simulink library "fm_copter_loiter_indi_lib"  (R2018b)
settings: Solver=VariableStepAuto  StartTime=0.0  StopTime=10.0  RelTol=1e-3
undefined symbols (not defined in the file or in its folder): fm_loiter
libraries: axes_transformation_lib x1, simulink x1, cntrl_horiz_pos_indi_lib x1, fm_copter_alt_hold_indi_lib x1
settings Model: Creator=Ybeyer  LastModifiedBy=Yannic
settings SFSimCC: SimUseLocalCustomCode=off
settings RTWCC: RTWUseLocalCustomCode=off
settings CodeAppCC: StateflowObjectComments=on

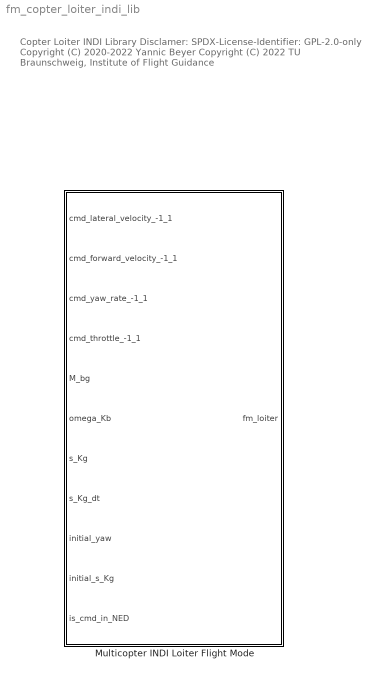
== system fm_copter_loiter_indi_lib ==
  note: Copter Loiter INDI Library
      |
      | Disclamer:
      | SPDX-License-Identifier: GPL-2.0-only
      |
      | Copyright (C) 2020-2022 Yannic Beyer
      | Copyright (C) 2022 TU Braunschweig, Institute of Flight Guidance
  Multicopter INDI Loiter Flight Mode : Subsystem  mask{fm=fm_loiter}
      mask prompts: fm "Multicopter INDI loiter flight  struct"
      mask DialogControl DescGroupVar Prompt: Multicopter INDI Loiter Flight Mode
      mask DialogControl DescTextVar Prompt: Loiter flight mode using the reduced attitude controller with INDI.
      mask DialogControl Control2 Prompt: To intialize the parameters struct see multicopterFlightModeLoiter.

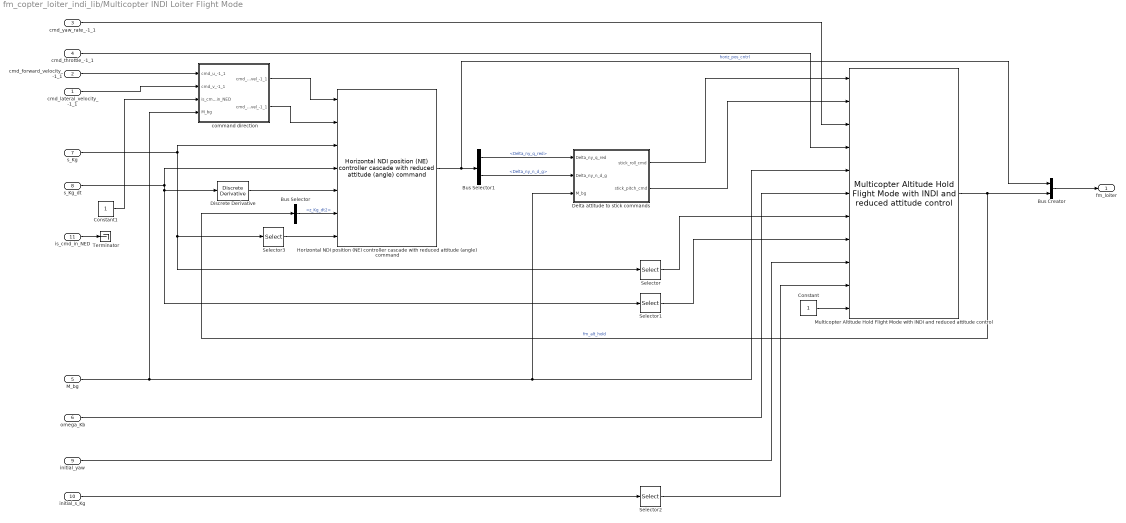
== system fm_copter_loiter_indi_lib/Multicopter INDI Loiter Flight Mode ==
  cmd_lateral_velocity_-1_1 : Inport  SampleTime=fm.sample_time
  cmd_forward_velocity_-1_1 : Inport  Port=2  SampleTime=fm.sample_time
  cmd_yaw_rate_-1_1 : Inport  Port=3  SampleTime=fm.sample_time
  cmd_throttle_-1_1 : Inport  Port=4  SampleTime=fm.sample_time
  M_bg : Inport  Port=5  SampleTime=fm.sample_time
  omega_Kb : Inport  Port=6  SampleTime=fm.sample_time
  s_Kg : Inport  Port=7  SampleTime=fm.sample_time
  s_Kg_dt : Inport  Port=8  SampleTime=fm.sample_time
  initial_yaw : Inport  Port=9  SampleTime=fm.sample_time
  initial_s_Kg : Inport  Port=10  SampleTime=fm.sample_time
  is_cmd_in_NED : Inport  Port=11  SampleTime=fm.sample_time
  Bus Creator : BusCreator  Inputs=2
  Bus Selector : BusSelector  OutputSignals=alt_cntrl.reference.z_Kg_dt2
  Bus Selector1 : BusSelector  OutputSignals=pseudo_control.Delta_ny_q_red,pseudo_control.Delta_ny_n_d_g
  Constant : Constant
  Constant1 : Constant  OutDataTypeStr=Inherit: Inherit via back propagation
  Delta attitude to stick commands : Subsystem
  Discrete Derivative : simulink/Discrete/Discrete Derivative  gainval=1.0  ICPrevScaledInput=0.0  OutMin=[]  OutMax=[]  OutDataType=fixdt(1, 16)  OutScaling=2^-10  DoSatur=off
  Horizontal NDI position (NE) controller cascade with reduced attitude (angle) command : cntrl_horiz_pos_indi_lib/Horizontal NDI position (NE) controller cascade with reduced attitude (angle) command  horiz_pos_cntrl=fm.horiz_pos_cntrl  T=2./fm.fm_alt.cntrl.atti_cntrl.rm.lean.omega + fm.fm_alt.motor_time_constant + 2./fm.fm_alt.sens_filt.omega
      settings: SourceProductName=LADAC
  Multicopter Altitude Hold Flight Mode with INDI and reduced attitude control : fm_copter_alt_hold_indi_lib/Multicopter Altitude Hold Flight Mode with INDI and reduced attitude control  fm=fm.fm_alt
      settings: SourceProductName=LADAC
  Selector : Selector  InputPortWidth=3  IndexOptions=Index vector (dialog)  Indices=3  OutputSizes=1
  Selector1 : Selector  InputPortWidth=3  IndexOptions=Index vector (dialog)  Indices=3  OutputSizes=1
  Selector2 : Selector  InputPortWidth=3  IndexOptions=Index vector (dialog)  Indices=3  OutputSizes=1
  Selector3 : Selector  InputPortWidth=3  IndexOptions=Index vector (dialog)  Indices=[1,2]  OutputSizes=1
  Terminator : Terminator
  command direction : Subsystem
  fm_loiter : Outport  OutDataTypeStr=single  SampleTime=fm.sample_time
  wires:
  cmd_forward_velocity_-1_1/1 -> command direction/1(cmd_u_-1_1)
  s_Kg_dt/1 -> Horizontal NDI position (NE) controller cascade with reduced attitude (angle) command/4, Discrete Derivative/1, Selector1/1
  Discrete Derivative/1 -> Horizontal NDI position (NE) controller cascade with reduced attitude (angle) command/5
  cmd_yaw_rate_-1_1/1 -> Multicopter Altitude Hold Flight Mode with INDI and reduced attitude control/3
  Constant/1 -> Multicopter Altitude Hold Flight Mode with INDI and reduced attitude control/11
  Selector3/1 -> Horizontal NDI position (NE) controller cascade with reduced attitude (angle) command/7
  initial_s_Kg/1 -> Selector2/1
  omega_Kb/1 -> Multicopter Altitude Hold Flight Mode with INDI and reduced attitude control/6
  Horizontal NDI position (NE) controller cascade with reduced attitude (angle) command/1 -> Bus Creator/1, Bus Selector1/1  "horiz_pos_cntrl"
  Bus Selector1/2 -> Delta attitude to stick commands/2(Delta_ny_n_d_g)  "<Delta_ny_n_d_g>"
  M_bg/1 -> Delta attitude to stick commands/3(M_bg), Multicopter Altitude Hold Flight Mode with INDI and reduced attitude control/5, command direction/4(M_bg)
  Multicopter Altitude Hold Flight Mode with INDI and reduced attitude control/1 -> Bus Creator/2, Bus Selector/1  "fm_alt_hold"
  Selector1/1 -> Multicopter Altitude Hold Flight Mode with INDI and reduced attitude control/8
  s_Kg/1 -> Horizontal NDI position (NE) controller cascade with reduced attitude (angle) command/3, Selector3/1, Selector/1
  Delta attitude to stick commands/2(stick_pitch_cmd) -> Multicopter Altitude Hold Flight Mode with INDI and reduced attitude control/2
  initial_yaw/1 -> Multicopter Altitude Hold Flight Mode with INDI and reduced attitude control/9
  cmd_throttle_-1_1/1 -> Multicopter Altitude Hold Flight Mode with INDI and reduced attitude control/4
  Bus Selector/1 -> Horizontal NDI position (NE) controller cascade with reduced attitude (angle) command/6  "<z_Kg_dt2>"
  cmd_lateral_velocity_-1_1/1 -> command direction/2(cmd_v_-1_1)
  Selector/1 -> Multicopter Altitude Hold Flight Mode with INDI and reduced attitude control/7
  Delta attitude to stick commands/1(stick_roll_cmd) -> Multicopter Altitude Hold Flight Mode with INDI and reduced attitude control/1
  Constant1/1 -> command direction/3(is_cmd_in_NED)
  Selector2/1 -> Multicopter Altitude Hold Flight Mode with INDI and reduced attitude control/10
  Bus Selector1/1 -> Delta attitude to stick commands/1(Delta_ny_q_red)  "<Delta_ny_q_red>"
  Bus Creator/1 -> fm_loiter/1
  command direction/1(cmd_north_vel_-1_1) -> Horizontal NDI position (NE) controller cascade with reduced attitude (angle) command/1
  command direction/2(cmd_east_vel_-1_1) -> Horizontal NDI position (NE) controller cascade with reduced attitude (angle) command/2
  is_cmd_in_NED/1 -> Terminator/1

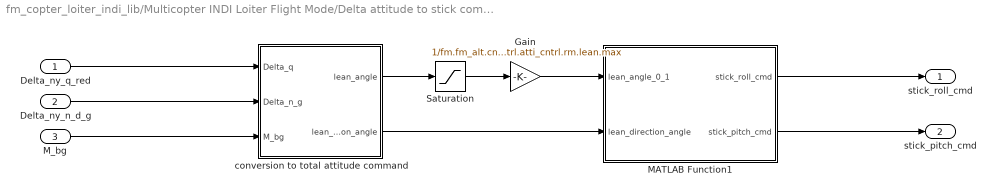
== system fm_copter_loiter_indi_lib/Multicopter INDI Loiter Flight Mode/Delta attitude to stick commands ==
  Delta_ny_q_red : Inport
  Delta_ny_n_d_g : Inport  Port=2
  M_bg : Inport  Port=3
  Gain : Gain  Gain=1/fm.fm_alt.cntrl.atti_cntrl.rm.lean.max
  MATLAB Function1 : MATLAB Function  TreatAsAtomicUnit=on
  Saturation : Saturate  UpperLimit=fm.fm_alt.cntrl.atti_cntrl.rm.lean.max  LowerLimit=0
  conversion to total attitude command : Subsystem
  stick_roll_cmd : Outport
  stick_pitch_cmd : Outport  Port=2
  wires:
  Saturation/1 -> Gain/1
  conversion to total attitude command/2(lean_direction_angle) -> MATLAB Function1/2(lean_direction_angle)
  conversion to total attitude command/1(lean_angle) -> Saturation/1
  MATLAB Function1/1(stick_roll_cmd) -> stick_roll_cmd/1
  MATLAB Function1/2(stick_pitch_cmd) -> stick_pitch_cmd/1
  Delta_ny_n_d_g/1 -> conversion to total attitude command/2(Delta_n_g)
  Delta_ny_q_red/1 -> conversion to total attitude command/1(Delta_q)
  M_bg/1 -> conversion to total attitude command/3(M_bg)
  Gain/1 -> MATLAB Function1/1(lean_angle_0_1)

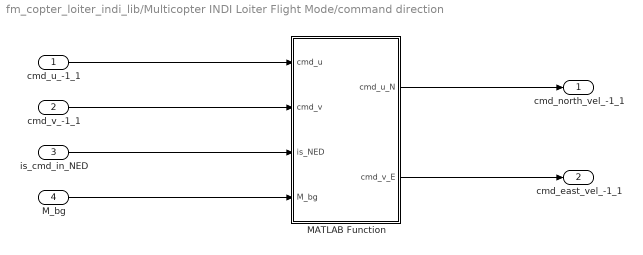
== system fm_copter_loiter_indi_lib/Multicopter INDI Loiter Flight Mode/command direction ==
  cmd_u_-1_1 : Inport
  cmd_v_-1_1 : Inport  Port=2
  is_cmd_in_NED : Inport  Port=3
  M_bg : Inport  Port=4
  MATLAB Function : MATLAB Function  TreatAsAtomicUnit=on
  cmd_north_vel_-1_1 : Outport
  cmd_east_vel_-1_1 : Outport  Port=2
  wires:
  cmd_u_-1_1/1 -> MATLAB Function/1(cmd_u)
  cmd_v_-1_1/1 -> MATLAB Function/2(cmd_v)
  is_cmd_in_NED/1 -> MATLAB Function/3(is_NED)
  MATLAB Function/1(cmd_u_N) -> cmd_north_vel_-1_1/1
  MATLAB Function/2(cmd_v_E) -> cmd_east_vel_-1_1/1
  M_bg/1 -> MATLAB Function/4(M_bg)

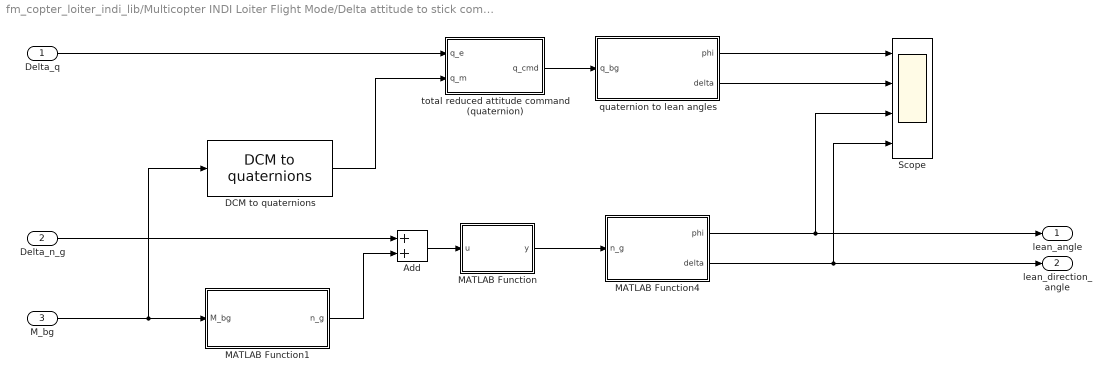
== system fm_copter_loiter_indi_lib/Multicopter INDI Loiter Flight Mode/Delta attitude to stick commands/conversion to total attitude command ==
  Delta_q : Inport
  Delta_n_g : Inport  Port=2
  M_bg : Inport  Port=3
  Add : Sum
  DCM to quaternions : axes_transformation_lib/DCM to quaternions  SystemSampleTime=-1
      settings: SourceProductName=LADAC
  MATLAB Function : MATLAB Function  TreatAsAtomicUnit=on
  MATLAB Function1 : MATLAB Function  TreatAsAtomicUnit=on
  MATLAB Function4 : MATLAB Function  TreatAsAtomicUnit=on
  Scope : Scope  NumInputPorts=4
  quaternion to lean angles : Subsystem
  total reduced attitude command (quaternion) : MATLAB Function  TreatAsAtomicUnit=on
  lean_angle : Outport
  lean_direction_angle : Outport  Port=2
  wires:
  MATLAB Function/1(y) -> MATLAB Function4/1(n_g)
  MATLAB Function1/1(n_g) -> Add/2
  Delta_n_g/1 -> Add/1
  MATLAB Function4/2(delta) -> lean_direction_angle/1, Scope/4
  quaternion to lean angles/2(delta) -> Scope/2
  MATLAB Function4/1(phi) -> Scope/3, lean_angle/1
  Delta_q/1 -> total reduced attitude command (quaternion)/1(q_e)
  Add/1 -> MATLAB Function/1(u)
  total reduced attitude command (quaternion)/1(q_cmd) -> quaternion to lean angles/1(q_bg)
  quaternion to lean angles/1(phi) -> Scope/1
  M_bg/1 -> DCM to quaternions/1, MATLAB Function1/1(M_bg)
  DCM to quaternions/1 -> total reduced attitude command (quaternion)/2(q_m)

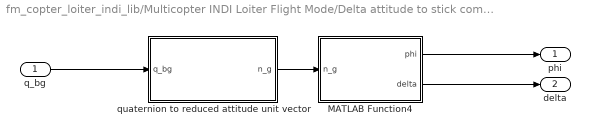
== system fm_copter_loiter_indi_lib/Multicopter INDI Loiter Flight Mode/Delta attitude to stick commands/conversion to total attitude command/quaternion to lean angles ==
  q_bg : Inport
  MATLAB Function4 : MATLAB Function  TreatAsAtomicUnit=on
  quaternion to reduced attitude unit vector : MATLAB Function  TreatAsAtomicUnit=on
  phi : Outport
  delta : Outport  Port=2
  wires:
  quaternion to reduced attitude unit vector/1(n_g) -> MATLAB Function4/1(n_g)
  MATLAB Function4/1(phi) -> phi/1
  q_bg/1 -> quaternion to reduced attitude unit vector/1(q_bg)
  MATLAB Function4/2(delta) -> delta/1

== matlab function fm_copter_loiter_indi_lib/Multicopter INDI Loiter Flight Mode/command direction/MATLAB Function ==
  data: cmd_u input; cmd_u_N output; cmd_v input; is_NED input; cmd_v_E output; M_bg input
function [cmd_u_N,cmd_v_E] = fcn( cmd_u, cmd_v, is_NED, M_bg )

if is_NED
    cmd_u_N = cmd_u;
    cmd_v_E = cmd_v;
else
    EulerAngle = dcm2Euler(M_bg);
    yaw = EulerAngle(3);
    M_NED_FRD = euler2Dcm([0;0;yaw])';
    cmd_V_NED = M_NED_FRD * [ cmd_u; cmd_v; 0 ];
    cmd_u_N = cmd_V_NED(1);
    cmd_v_E = cmd_V_NED(2);
end

end

== matlab function fm_copter_loiter_indi_lib/Multicopter INDI Loiter Flight Mode/Delta attitude to stick commands/conversion to total attitude command/MATLAB Function1 ==
  data: M_bg input; n_g output
function n_g = dcm2LeanVector( M_bg )
n_g = dcm2LeanVector( M_bg );
end

== matlab function fm_copter_loiter_indi_lib/Multicopter INDI Loiter Flight Mode/Delta attitude to stick commands/MATLAB Function1 ==
  data: lean_angle_0_1 input; stick_roll_cmd output; lean_direction_angle input; stick_pitch_cmd output
function [stick_roll_cmd,stick_pitch_cmd] = fcn(lean_angle_0_1,lean_direction_angle)

stick_roll_cmd = lean_angle_0_1 * sin( lean_direction_angle );
stick_pitch_cmd = - lean_angle_0_1 * cos( lean_direction_angle );

end

== matlab function fm_copter_loiter_indi_lib/Multicopter INDI Loiter Flight Mode/Delta attitude to stick commands/conversion to total attitude command/MATLAB Function ==
  data: u input; y output
function y = fcn(u)

y = u/norm(u,2);

== matlab function fm_copter_loiter_indi_lib/Multicopter INDI Loiter Flight Mode/Delta attitude to stick commands/conversion to total attitude command/MATLAB Function4 ==
  data: n_g input; phi output; delta output
function [phi,delta] = fcn(n_g)

phi = acos( max( -1, min( 1, -n_g(3) ) ) );

delta = atan2(n_g(2),n_g(1));

== matlab function fm_copter_loiter_indi_lib/Multicopter INDI Loiter Flight Mode/Delta attitude to stick commands/conversion to total attitude command/quaternion to lean angles/MATLAB Function4 ==
  data: n_g input; phi output; delta output
function [phi,delta] = fcn(n_g)

phi = acos( max( -1, min( 1, -n_g(3) ) ) );

delta = atan2(n_g(2),n_g(1));

== matlab function fm_copter_loiter_indi_lib/Multicopter INDI Loiter Flight Mode/Delta attitude to stick commands/conversion to total attitude command/quaternion to lean angles/quaternion to reduced attitude unit vector ==
  data: q_bg input; n_g output
function n_g = fcn( q_bg )
M_bg = quat2Dcm(q_bg);
n_g = dcm2LeanVector( M_bg );
end

== matlab function fm_copter_loiter_indi_lib/Multicopter INDI Loiter Flight Mode/Delta attitude to stick commands/conversion to total attitude command/total reduced attitude command (quaternion) ==
  data: q_e input; q_m input; q_cmd output
function q_cmd = fcn(q_e, q_m)

q_cmd = quatMultiply( q_m, q_e );
